simulink model "Waveformmodel"  (R2021b)
settings: Solver=FixedStepAuto  StartTime=0.0  StopTime=1  FixedStep=0.001  RelTol=1e-3
undefined symbols (not defined in the file or in its folder): pAmpGain, pClampAmpl, pClampOffs, pClampSatMax, pClampSatMin, pShearAmpl, pShearOffs, pShearSatMax, pShearSatMin
libraries: simulink x2
settings Model: Creator=20191779  LastModifiedBy=20191777

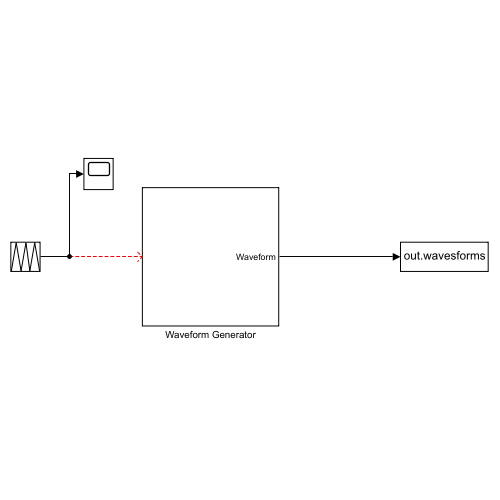
[thumbnail: Simulink's stored preview of the top-level diagram]
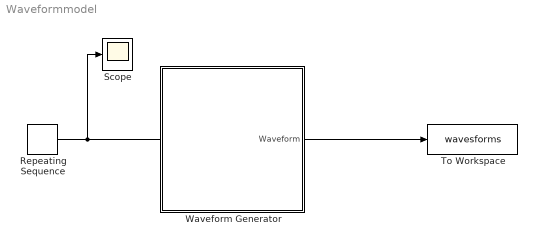
== system Waveformmodel ==
  Repeating Sequence : simulink/Sources/Repeating Sequence  rep_seq_t=[0 1 2]  rep_seq_y=[0 5 0]*5e-6
  Scope : Scope
  To Workspace : ToWorkspace  VariableName=wavesforms  SampleTime=-1
  Waveform Generator : Subsystem
  wires:
  Repeating Sequence/1 -> Scope/1
  Waveform Generator/1(Waveform) -> To Workspace/1

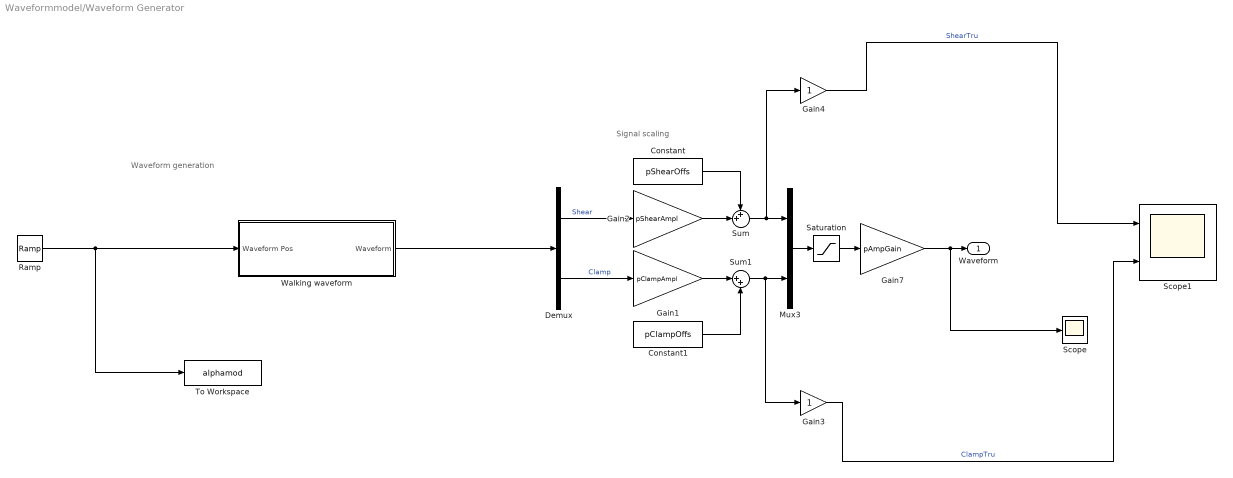
== system Waveformmodel/Waveform Generator ==
  note: Waveform generation
  note: Signal scaling
  Constant : Constant  Value=pShearOffs
  Constant1 : Constant  Value=pClampOffs
  Demux : Demux  Outputs=2
  Gain1 : Gain  Gain=pClampAmpl
  Gain2 : Gain  Gain=pShearAmpl
  Gain3 : Gain
  Gain4 : Gain
  Gain7 : Gain  Gain=pAmpGain
  Mux3 : Mux  Inputs=2
  Ramp : simulink/Sources/Ramp  slope=2*pi  start=0  InitialOutput=0
  Saturation : Saturate  UpperLimit=[pShearSatMax pShearSatMax pClampSatMax pClampSatMax]  LowerLimit=[pShearSatMin pShearSatMin pClampSatMin pClampSatMin]
  Scope : Scope
  Scope1 : Scope  NumInputPorts=2
  Sum : Sum  Inputs=++|
  Sum1 : Sum  Inputs=|++
  To Workspace : ToWorkspace  VariableName=alphamod  SampleTime=-1
  Walking waveform : Subsystem  TreatAsAtomicUnit=on
  Waveform : Outport  VectorParamsAs1DForOutWhenUnconnected=off
  wires:
  Gain2/1 -> Sum/2
  Constant/1 -> Sum/1
  Gain1/1 -> Sum1/1
  Constant1/1 -> Sum1/2
  Demux/1 -> Gain2/1  "Shear"
  Demux/2 -> Gain1/1  "Clamp"
  Gain3/1 -> Scope1/2  "ClampTru"
  Gain4/1 -> Scope1/1  "ShearTru"
  Walking waveform/1(Waveform) -> Demux/1
  Mux3/1 -> Saturation/1
  Gain7/1 -> Scope/1, Waveform/1
  Sum/1 -> Gain4/1, Mux3/1
  Sum1/1 -> Gain3/1, Mux3/2
  Saturation/1 -> Gain7/1
  Ramp/1 -> To Workspace/1, Walking waveform/1(Waveform Pos)

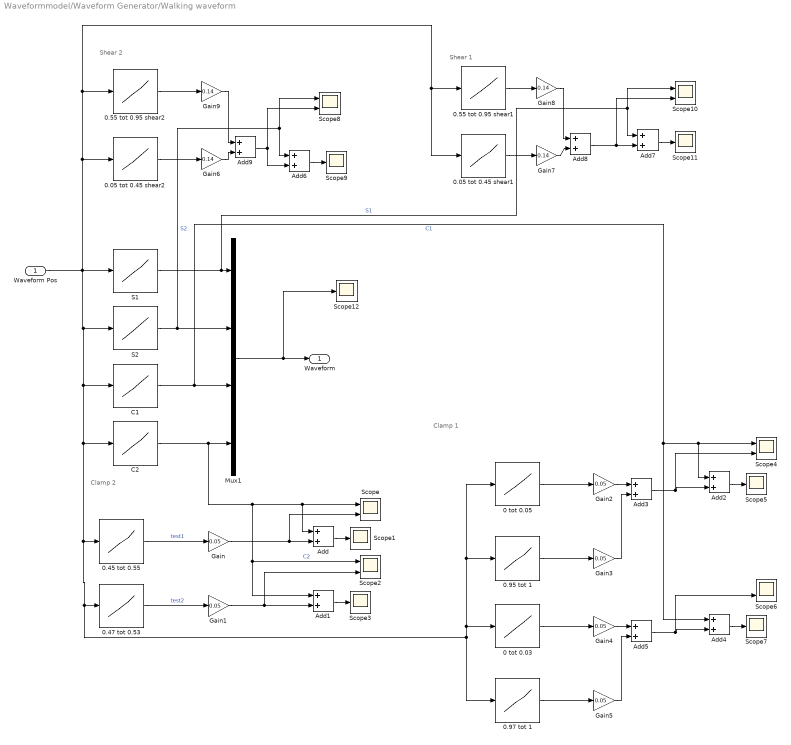
== system Waveformmodel/Waveform Generator/Walking waveform ==
  note: Shear 1
  note: Shear 2
  note: Clamp 2
  note: Clamp 1
  Waveform Pos : Inport
  0 tot 0.03 : Lookup_n-D  NumberOfTableDimensions=1  BreakpointsForDimension1="[0.45*2*pi, 0.5*2*pi,  0.55*2*pi]-pi"  Table=[0, -1, 0]  InterpMethod=Cubic spline  ExtrapMethod=Clip  InternalRulePriority=Speed  RndMeth=Simplest  InputSameDT=on
  0 tot 0.05 : Lookup_n-D  NumberOfTableDimensions=1  BreakpointsForDimension1="[0.45*2*pi, 0.5*2*pi,  0.55*2*pi]-pi"  Table=[0, -1, 0]  InterpMethod=Cubic spline  ExtrapMethod=Clip  InternalRulePriority=Speed  RndMeth=Simplest  InputSameDT=on
  0.05 tot 0.45 shear1 : Lookup_n-D  NumberOfTableDimensions=1  BreakpointsForDimension1="[0.05*2*pi, 0.15*2*pi, 0.25*2*pi,  0.35*2*pi, 0.45*2*pi]"  Table=[0, 1, 0, -1, 0]  InterpMethod=Cubic spline  ExtrapMethod=Clip  InternalRulePriority=Speed  RndMeth=Simplest  InputSameDT=on
  0.05 tot 0.45 shear2 : Lookup_n-D  NumberOfTableDimensions=1  BreakpointsForDimension1="[0.05*2*pi, 0.15*2*pi, 0.25*2*pi,  0.35*2*pi, 0.45*2*pi]"  Table=[0, 1, 0, -1, 0]  InterpMethod=Cubic spline  ExtrapMethod=Clip  InternalRulePriority=Speed  RndMeth=Simplest  InputSameDT=on
  0.45 tot 0.55 : Lookup_n-D  NumberOfTableDimensions=1  BreakpointsForDimension1="[0.45*2*pi, 0.5*2*pi,  0.55*2*pi]"  Table=[0, -1, 0]  InterpMethod=Cubic spline  ExtrapMethod=Clip  InternalRulePriority=Speed  RndMeth=Simplest  InputSameDT=on
  0.47 tot 0.53 : Lookup_n-D  NumberOfTableDimensions=1  BreakpointsForDimension1="[0.47*2*pi, 0.5*2*pi,  0.53*2*pi]"  Table=[0, -1, 0]  InterpMethod=Cubic spline  ExtrapMethod=Clip  InternalRulePriority=Speed  RndMeth=Simplest  InputSameDT=on
  0.55 tot 0.95 shear1 : Lookup_n-D  NumberOfTableDimensions=1  BreakpointsForDimension1="[0.05*2*pi, 0.15*2*pi, 0.25*2*pi,  0.35*2*pi, 0.45*2*pi]+pi"  Table=[0, 1, 0, -1, 0]  InterpMethod=Cubic spline  ExtrapMethod=Clip  InternalRulePriority=Speed  RndMeth=Simplest  InputSameDT=on
  0.55 tot 0.95 shear2 : Lookup_n-D  NumberOfTableDimensions=1  BreakpointsForDimension1="[0.05*2*pi, 0.15*2*pi, 0.25*2*pi,  0.35*2*pi, 0.45*2*pi]+pi"  Table=[0, 1, 0, -1, 0]  InterpMethod=Cubic spline  ExtrapMethod=Clip  InternalRulePriority=Speed  RndMeth=Simplest  InputSameDT=on
  0.95 tot 1 : Lookup_n-D  NumberOfTableDimensions=1  BreakpointsForDimension1="[0.45*2*pi, 0.5*2*pi,  0.55*2*pi]+pi"  Table=[0, -1, 0]  InterpMethod=Cubic spline  ExtrapMethod=Clip  InternalRulePriority=Speed  RndMeth=Simplest  InputSameDT=on
  0.97 tot 1 : Lookup_n-D  NumberOfTableDimensions=1  BreakpointsForDimension1="[0.45*2*pi, 0.5*2*pi,  0.55*2*pi]+pi"  Table=[0, -1, 0]  InterpMethod=Cubic spline  ExtrapMethod=Clip  InternalRulePriority=Speed  RndMeth=Simplest  InputSameDT=on
  Add{,1..9} (10 alike) : Sum
  C1 : Lookup_n-D  NumberOfTableDimensions=1  BreakpointsForDimension1=[0, 0.05*2*pi, 0.45*2*pi, 0.55*2*pi, 0.95*2*pi, 1*2*pi]  Table=[1, 1, -1, -1, 1, 1]  InternalRulePriority=Speed  RndMeth=Simplest  InputSameDT=on
  C2 : Lookup_n-D  NumberOfTableDimensions=1  BreakpointsForDimension1=[0, 0.05*2*pi, 0.45*2*pi, 0.55*2*pi, 0.95*2*pi, 1*2*pi]  Table=[-1, -1, 1, 1, -1, -1]  InternalRulePriority=Speed  RndMeth=Simplest  InputSameDT=on
  Gain{,1..5} (6 alike) : Gain  Gain=0.05
  Gain{6..9} (4 alike) : Gain  Gain=0.14
  Mux1 : Mux
  S1 : Lookup_n-D  NumberOfTableDimensions=1  BreakpointsForDimension1=[0, 0.45*2*pi, 0.55*2*pi, 1*2*pi]  Table=[0, 1, -1, 0]  InternalRulePriority=Speed  RndMeth=Simplest  InputSameDT=on
  S2 : Lookup_n-D  NumberOfTableDimensions=1  BreakpointsForDimension1=[0, 0.05*2*pi, 0.95*2*pi, 1*2*pi]  Table=[0, -1, 1, 0]  InternalRulePriority=Speed  RndMeth=Simplest  InputSameDT=on
  Scope{,2,4,6,8,10} (6 alike) : Scope  NumInputPorts=2
  Scope{1,3,5,7,9,11..12} (7 alike) : Scope
  Waveform : Outport  VectorParamsAs1DForOutWhenUnconnected=off
  wires:
  Mux1/1 -> Scope12/1, Waveform/1
  0.45 tot 0.55/1 -> Gain/1  "test1"
  Gain/1 -> Scope/2, Add/2
  Add/1 -> Scope1/1
  0.47 tot 0.53/1 -> Gain1/1  "test2"
  Add1/1 -> Scope3/1
  C2/1 -> Mux1/4, Add1/1, Scope2/1, Add/1, Scope/1  "C2"
  Gain1/1 -> Add1/2, Scope2/2
  Add2/1 -> Scope5/1
  0 tot 0.05/1 -> Gain2/1
  0.95 tot 1/1 -> Gain3/1
  Gain2/1 -> Add3/1
  Add3/1 -> Add2/2, Scope4/2
  Gain3/1 -> Add3/2
  Gain5/1 -> Add5/2
  Add5/1 -> Add4/2, Scope6/2
  C1/1 -> Mux1/3, Add4/1, Add2/1, Scope4/1  "C1"
  Gain4/1 -> Add5/1
  0 tot 0.03/1 -> Gain4/1
  Add4/1 -> Scope7/1
  0.97 tot 1/1 -> Gain5/1
  Add6/1 -> Scope9/1
  S2/1 -> Add6/1, Scope8/1, Mux1/2  "S2"
  0.05 tot 0.45 shear2/1 -> Gain6/1
  0.05 tot 0.45 shear1/1 -> Gain7/1
  S1/1 -> Mux1/1, Add7/1, Scope10/1  "S1"
  Add7/1 -> Scope11/1
  Gain7/1 -> Add8/2
  0.55 tot 0.95 shear1/1 -> Gain8/1
  Add8/1 -> Scope10/2, Add7/2
  Gain8/1 -> Add8/1
  0.55 tot 0.95 shear2/1 -> Gain9/1
  Waveform Pos/1 -> 0.55 tot 0.95 shear2/1, 0.05 tot 0.45 shear1/1, 0.55 tot 0.95 shear1/1, 0.05 tot 0.45 shear2/1, C2/1, 0 tot 0.05/1, 0.95 tot 1/1, 0 tot 0.03/1, 0.97 tot 1/1, 0.47 tot 0.53/1, 0.45 tot 0.55/1, C1/1, S2/1, S1/1
  Gain6/1 -> Add9/2
  Gain9/1 -> Add9/1
  Add9/1 -> Scope8/2, Add6/2
